simulink model "Modelo"  (R2021b)
settings: Solver=FixedStepDiscrete  StartTime=0.0  StopTime=inf  FixedStep=0.002  RelTol=1e-3  EnableMultiTasking=on
undefined symbols (not defined in the file): Jeq, km, kt, Rm
settings Model: ExtModeTrigDuration=10000  Creator=ricar  LastModifiedBy=ricar
settings SolverCC: AlgebraicLoopSolver=TrustRegion  PositivePriorityOrder=on
settings DataIOCC: ReturnWorkspaceOutputs=off
settings DebuggingCC: SFMachineParentedDataDiag=warning  ArithmeticOperatorsInVariantConditions=warning
settings SFSimCC: SimUseLocalCustomCode=off  CustomCodeUndefinedFunction=UseInterfaceOnly
settings RTWCC: Description=QUARC Win64 Target Using Toolchain  SystemTargetFile=quarc_win64.tlc  TemplateMakefile=quarc_default_tmf  RTWUseLocalCustomCode=off  Toolchain=QUARC win64 | nmake (64-bit Windows)  BuildConfiguration=Faster Runs
settings CodeAppCC: StateflowObjectComments=on
settings STFCustomTargetCC: TargetLangStandard=C99 (ISO)  ConcurrentExecutionCompliant=on  UseToolchainInfoCompliant=on  SystemTargetFile=quarc_win64.tlc
settings GRTTargetCC: ParMdlRefBuildCompliant=off  CompOptLevelCompliant=off  CombineOutputUpdateFcns=off  MatFileLogging=off  CPPClassGenCompliant=off  GRTInterface=on  ExtMode=on  ExtModeMexFile=quarc_comm
settings ConfigComp: CovMetricSettings=dswe

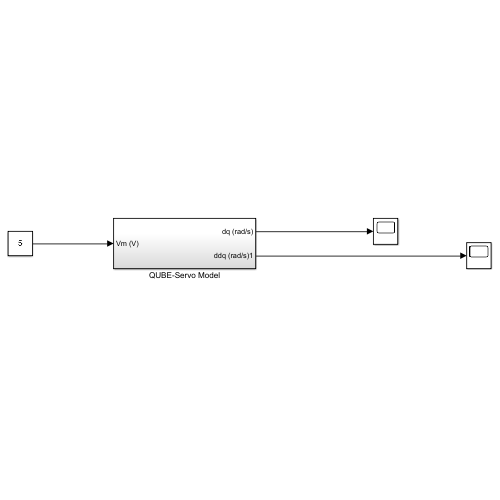
[thumbnail: Simulink's stored preview of the top-level diagram]
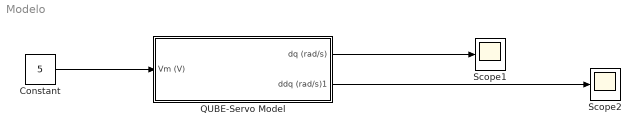
== system Modelo ==
  Constant : Constant  Value=5
  QUBE-Servo Model : Subsystem
  Scope1 : Scope
  Scope2 : Scope
  wires:
  Constant/1 -> QUBE-Servo Model/1(Vm (V))
  QUBE-Servo Model/2(ddq (rad/s)1) -> Scope2/1
  QUBE-Servo Model/1(dq (rad/s)) -> Scope1/1

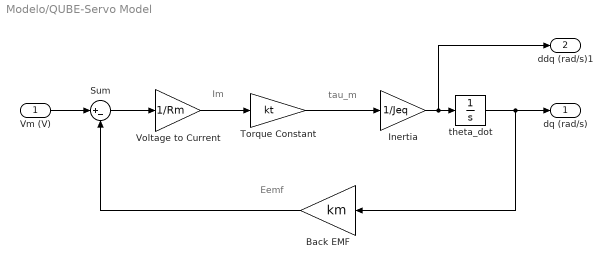
== system Modelo/QUBE-Servo Model ==
  note: Im
  note: tau_m
  note: Eemf
  Vm (V) : Inport
  Back EMF : Gain  Gain=km  SaturateOnIntegerOverflow=on  OutDataTypeStr=Inherit: Same as input  ParamDataTypeStr=Inherit: Same as input
  Inertia : Gain  Gain=1/Jeq  SaturateOnIntegerOverflow=on  OutDataTypeStr=Inherit: Same as input  ParamDataTypeStr=Inherit: Same as input
  Sum : Sum  Inputs=|+-  InputSameDT=on  SaturateOnIntegerOverflow=on  OutDataTypeStr=Inherit: Same as first input
  Torque Constant : Gain  Gain=kt
  Voltage to Current : Gain  Gain=1/Rm  SaturateOnIntegerOverflow=on  OutDataTypeStr=Inherit: Same as input  ParamDataTypeStr=Inherit: Same as input
  theta_dot : Integrator
  dq (rad/s) : Outport
  ddq (rad/s)1 : Outport  Port=2
  wires:
  Voltage to Current/1 -> Torque Constant/1
  Vm (V)/1 -> Sum/1
  Sum/1 -> Voltage to Current/1
  theta_dot/1 -> Back EMF/1, dq (rad/s)/1
  Torque Constant/1 -> Inertia/1
  Inertia/1 -> ddq (rad/s)1/1, theta_dot/1
  Back EMF/1 -> Sum/2
